simulink model "stm32f4_input_debounce"  (Simulink 7.3)
settings: Solver=FixedStepDiscrete  StartTime=0.0  StopTime=1  RelTol=1e-3
libraries: simulink x3, stm32f4_io_lib x1
settings Model: Creator=Krisada  LastModifiedBy=Krisada

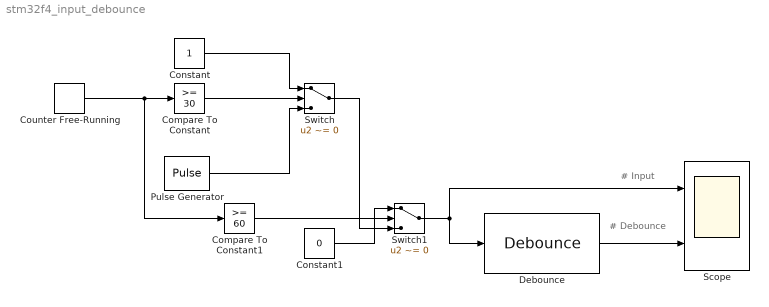
== system stm32f4_input_debounce ==
  note: # Input
  note: # Debounce
  Compare To Constant : simulink/Logic and Bit Operations/Compare To Constant  SystemSampleTime=-1  relop=>=  const=30  LogicOutDataTypeMode=uint8  ZeroCross=off
  Compare To Constant1 : simulink/Logic and Bit Operations/Compare To Constant  SystemSampleTime=-1  relop=>=  const=60  LogicOutDataTypeMode=uint8  ZeroCross=off
  Constant : Constant  OutDataType=fixdt(1, 16)  OutScaling=2^0  SampleTime=0.01
  Constant1 : Constant  Value=0  OutDataType=fixdt(1, 16)  OutScaling=2^0  SampleTime=0.01
  Counter Free-Running : simulink/Sources/Counter Free-Running  SystemSampleTime=-1  NumBits=32  tsamp=0.01
  Debounce : stm32f4_io_lib/Debounce  SystemSampleTime=-1  mode=Toggle Latch  prescale=16  debounce=16
  Pulse Generator : DiscretePulseGenerator  PulseType=Time based  Amplitude=1  Period=0.02  PulseWidth=50  PhaseDelay=0  SampleTime=1
  Scope : Scope  NumInputPorts=2
      settings: YMin=-2~-2  YMax=2~2  SampleInput=on
  Switch : Switch  Criteria=u2 ~= 0  OutDataType=fixdt(1, 16)  OutScaling=2^0  SampleTime=0.01
  Switch1 : Switch  Criteria=u2 ~= 0  OutDataType=fixdt(1, 16)  OutScaling=2^0  SampleTime=0.01
  wires:
  Pulse Generator/1 -> Switch/3
  Constant/1 -> Switch/1
  Counter Free-Running/1 -> Compare To Constant/1, Compare To Constant1/1
  Compare To Constant1/1 -> Switch1/2
  Switch/1 -> Switch1/3
  Constant1/1 -> Switch1/1
  Switch1/1 -> Debounce/1, Scope/1
  Compare To Constant/1 -> Switch/2
  Debounce/1 -> Scope/2
